simulink model "t6_recurso3"  (R2024a)
settings: Solver=ode4  StartTime=0.0  StopTime=20  FixedStep=0.01  RelTol=1e-6  AbsTol=1e-6
InitFcn:
  | %wn = 10;
  | %xi = 0;
undefined symbols (not defined in the file): wn, xi
settings Model: Creator=scpmoxxa  LastModifiedBy=scpmoxxa
settings DataIOCC: SaveFormat=Array  SaveState=on
settings OptimizationCC: ReuseModelBlockBuffer=off
settings RTWCC: GPUComputeCapability=3.5

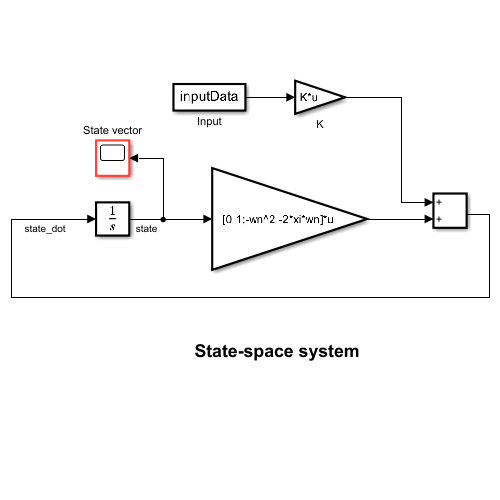
[thumbnail: Simulink's stored preview of the top-level diagram]
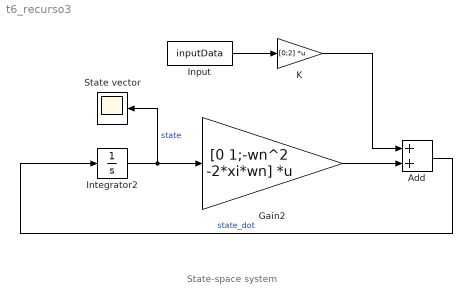
== system t6_recurso3 ==
  note: State-space system
  Add : Sum
  Gain2 : Gain  Gain=[0 1;-wn^2 -2*xi*wn]  Multiplication=Matrix(K*u)
  Input : FromWorkspace  VariableName=inputData
  Integrator2 : Integrator  InitialCondition=[1;0]
  K : Gain  Gain=[0;2]  Multiplication=Matrix(K*u)
  State vector : Scope
  wires:
  Integrator2/1 -> State vector/1, Gain2/1  "state"
  K/1 -> Add/1
  Gain2/1 -> Add/2
  Add/1 -> Integrator2/1  "state_dot"
  Input/1 -> K/1
